simulink model "SIM_EXO_DAL"  (R2021b)
settings: Solver=VariableStepAuto  StartTime=0.0  StopTime=60  FixedStep=0.0001  RelTol=1e-4
undefined symbols (not defined in the file): b, dq, q, X, Y, Z
libraries: sm_lib x47, nesl_utility x7
(part 19 of 25)

== matlab function SIM_EXO_DAL/Exoesqueleto/Dinámica Directa/D_dq ==
  data: b input; D_dq output; dq input
function D_dq = D_dq(b,dq)
%#codegen

%    This function was generated by the Symbolic Math Toolbox version 9.0.
%    02-Dec-2021 21:08:09
be = 5.02e-6;
if b(1) == 0
    be = 0;
end
b1 = b(1)+be;
b2 = b(2)+be;
b3 = b(3)+be;
b4 = b(4)+be;
b5 = b(5)+be;
b6 = b(6)+be;

dq1 = dq(1);
dq2 = dq(2);
dq3 = dq(3);
dq4 = dq(4);
dq5 = dq(5);
dq6 = dq(6);

D_dq = [b1.*dq1;b2.*dq2;b3.*dq3;b4.*dq4;b5.*dq5;b6.*dq6];

== matlab function SIM_EXO_DAL/Energy Analysis/P ==
  data: q input; P output
function P = P(q)
%#codegen
q1 = q(1);
q2 = q(2);
q3 = q(3);
q4 = q(4);
q5 = q(5);
q6 = q(6);
%    This function was generated by the Symbolic Math Toolbox version 9.0.
%    02-Dec-2021 21:38:45

t2 = cos(q4);
t3 = cos(q5);
t4 = cos(q6);
t5 = sin(q4);
t6 = sin(q5);
t7 = sin(q6);
t8 = q1+q2;
t14 = 9.007199254740992e+15;
t9 = cos(t8);
t10 = sin(t8);
t16 = (q3.*t14)./9.007199254740992e+15;
t11 = t10.*4.602992943936994e+15;
t12 = t9.*7.742227997977903e+15;
t17 = cos(t16);
t18 = sin(t16);
t13 = -t11;
t19 = t17.*7.38843356682345e-1;
t20 = t17.*2.61156643317655e-1;
t21 = t17.*4.392651260556773e-1;
t22 = t2.*t14.*t18.*(t11-t12).*(-1.232595164407831e-32);
t23 = t5.*t14.*t18.*(t11-t12).*(-1.232595164407831e-32);
t24 = (t5.*t14.*t18.*(t11-t12))./8.112963841460668e+31;
t15 = t12+t13;
t25 = t19+2.61156643317655e-1;
t26 = t20+7.38843356682345e-1;
t27 = t21-4.392651260556773e-1;
t28 = t9.*t25;
t29 = t10.*t26;
t30 = t9.*t27;
t31 = t10.*t27;
t32 = -t29;
t33 = -t31;
t36 = -t2.*(t29-t30);
t38 = -t5.*(t29-t30);
t41 = -t6.*(t5.*(t29-t30)+(t2.*t14.*t18.*(t11-t12))./8.112963841460668e+31);
t34 = t30+t32;
t35 = t28+t33;
t39 = t22+t38;
t40 = t24+t36;
t37 = t3.*t35;
t42 = t37+t41;
et1 = t9.*3.412222012061753e-3;
et2 = t10.*5.313226374396773e-3;
et3 = t4.*(t23+t2.*(t29-t30)).*7.125499486421585e-4-t7.*(t23+t2.*(t29-t30)).*1.31098465253029e-3;
et4 = 3.963167671901972e+15.*cos(q1+atan(3.077527609784337e-1)).*1.978770022836862e-18;
et5 = t3.*t9.*1.11711378834605e-4;
et6 = t3.*t10.*1.878983903386652e-4;
et7 = t9.*t17.*3.021813293822463e-3;
et8 = t10.*t17.*(-1.796561051029836e-3);
et9 = t6.*t35.*(-1.37594917755e-10)+t4.*t42.*1.31098465253029e-3;
et10 = t7.*t42.*7.125499486421585e-4;
et11 = t3.*(t5.*(t29-t30)+(t2.*t14.*t18.*(t11-t12))./8.112963841460668e+31).*(-1.37594917755e-10);
et12 = t5.*t6.*t9.*(-1.878983903386652e-4);
et13 = t5.*t6.*t10.*(-3.16044842165395e-4);
et14 = t3.*t9.*t17.*3.16044842165395e-4;
et15 = t3.*t10.*t17.*(-1.878983903386652e-4);
et16 = t5.*t6.*t9.*t17.*1.878983903386652e-4;
et17 = t5.*t6.*t10.*t17.*(-1.11711378834605e-4)+t2.*t6.*t9.*t14.*t18.*4.082091644006594e-20;
et18 = t2.*t6.*t10.*t14.*t18.*(-2.426929178367519e-20);
P = et1+et2+et3+et4+et5+et6+et7+et8+et9+et10+et11+et12+et13+et14+et15+et16+et17+et18;
